simulink model "sf_demo_tl30"  (Simulink 7.5)
settings: Solver=FixedStepDiscrete  StartTime=0.0  StopTime=20  FixedStep=0.5  RelTol=1e-3
PreLoadFcn:
  | if exist('tl_preloadfcn','file'), tl_preloadfcn(gcs,101); end
PostLoadFcn:
  | if exist('tl_postloadfcn','file'), tl_postloadfcn(gcs,101); end
InitFcn:
  | if exist('tlds_init','file'), tlds_init(gcs); end
StartFcn:
  | if exist('tlds_start','file'), tlds_start(gcs); end
StopFcn:
  | if exist('tlds_stop','file'), tlds_stop(gcs); end
undefined symbols (not defined in the file or in its folder): slDataTypeAndScale
libraries: tllib x6
PreSaveFcn:
  | if exist('tl_presavefcn','file'), tl_presavefcn(gcs); end
settings Model: DS_PROJECTFILE=sf_demo_tl30.dd  TL_MAIN_DATA={'#advcodeopt',0,'codeopt',{'inliningthreshold',5,'assembler',1,'optlevel',0,'decimals',0},'frameopt',{'mexargs',''},'logopt',{'plotinterval',0.1,'globalloggingmode',4},'date',735991.66639069444}  TL_MODEL_COMMENT=This model implements a simple state machine.  TLRevision=101  Creator=rwilts  LastModifiedBy=alex  ExtModeTrigMode=oneshot  ExtModeArmWhenConnect=off  BufferReuse=off
settings DataIOCC: LimitDataPoints=off
settings OptimizationCC: BlockReduction=off  BooleanDataType=off  OptimizeBlockIOStorage=off  BufferReuse=off  ExpressionFolding=off  LocalBlockOutputs=off  InitFltsAndDblsToZero=on
settings DebuggingCC: SaveWithParameterizedLinksMsg=none  SignalResolutionControl=TryResolveAllWithWarning  SolverPrmCheckMsg=none  MultiTaskDSMMsg=warning  MultiTaskCondExecSysMsg=none
settings HardwareCC: TargetEndianess=LittleEndian  TargetHWDeviceType=MATLAB Host  ProdEqTarget=off
settings RTWCC: IncludeERTFirstTime=on
settings GRTTargetCC: TargetFcnLib=ansi_tfl_tmw.mat

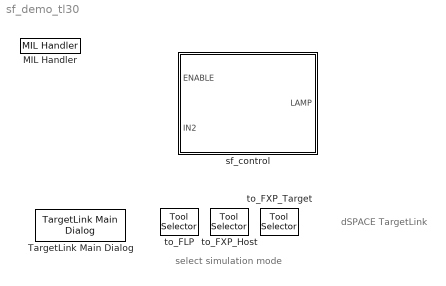
== system sf_demo_tl30 ==
  note: select simulation mode
  note: dSPACE TargetLink
  MIL Handler : tllib/MIL Handler  data={'date',735991.66638890048}
  TargetLink Main Dialog : tllib/TargetLink Main Dialog  SystemSampleTime=-1
  sf_control : Subsystem  Tag=TargetLink Simulation Frame
      settings: CopyFcn=if exist('tl_copyfcn','file'), tl_copyfcn(gcbh); end  NameChangeFcn=if exist('tl_framenamechangefcn','file'), tl_framenamechangefcn(gcbh); end
      settings: OpenFcn=|
      | if exist('open_tlsubsystem','file')
      |    open_tlsubsystem(gcbh);
      | else
      |    tlsubsystem = ...
      |       find_system(gcb, ...
      |       'LookUnderMasks','on', ...
      |       'FollowLinks','on', ...
      |       'Tag','MIL Subsystem');
      |    open_system(tlsubsystem);
      | end
      mask Type: TL_SimFrame
      mask Display: disp('TargetLink\nModel-\nin-the-loop\nmode')
  to_FLP : tllib/Tool Selector  Description=MIL\nmode  SystemSampleTime=-1  data={'date',735991.66638510418}
  to_FXP_Host : tllib/Tool Selector  Description=SIL\nmode  SystemSampleTime=-1  data={'date',735991.66638506949}
  to_FXP_Target : tllib/Tool Selector  Description=PIL\nmode  SystemSampleTime=-1  data={'date',735991.66638503468}

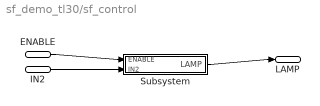
== system sf_demo_tl30/sf_control ==
  ENABLE : Inport  SampleTime=0.5  DataType=Specify via dialog  OutDataType=slDataTypeAndScale(('osc_int16'),('2^0'))  OutDataTypeStr=slDataTypeAndScale(('osc_int16'),('2^0'))
  IN2 : Inport  Port=2  SampleTime=0.5  DataType=Specify via dialog  OutDataType=osc_int16  OutDataTypeStr=osc_int16
  Subsystem : Subsystem  Tag=struct('sfcnName','sf_control_sf','subFunction','','srcSubsystem','')
      settings: OpenFcn=warndlg(get_param(gcb,'MaskHelp'),'Serious Warning');
      mask Type: TL_Enable
      mask Help: This subsystem keeps the TargetLink subsystem (subsystem with TargetLink blocks for production code generation), and is needed for the TargetLink simulation frame to work properly. DO NOT DELETE OR MODIFY IT!
  LAMP : Outport  OutDataType=sfix(16)  OutScaling=2^0
  wires:
  ENABLE/1 -> Subsystem/1(ENABLE)
  IN2/1 -> Subsystem/2(IN2)
  Subsystem/1(LAMP) -> LAMP/1

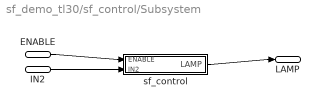
== system sf_demo_tl30/sf_control/Subsystem ==
  ENABLE : Inport  SampleTime=0.5  DataType=Specify via dialog  OutDataType=slDataTypeAndScale(('osc_int16'),('2^0'))  OutDataTypeStr=slDataTypeAndScale(('osc_int16'),('2^0'))
  IN2 : Inport  Port=2  SampleTime=0.5  DataType=Specify via dialog  OutDataType=osc_int16  OutDataTypeStr=osc_int16
  sf_control : Subsystem  Tag=MIL Subsystem  Description=a
      settings: CopyFcn=if exist('tl_copyfcn','file'), tl_copyfcn(gcbh); end  NameChangeFcn=if exist('tl_namechangefcn','file'), tl_namechangefcn(gcbh); end  DestroyFcn=if exist('update_tl_main_dlg','file'), update_tl_main_dlg('TL_subs_display'); end
      mask Display: disp('TargetLink Subsystem')
  LAMP : Outport  OutDataType=sfix(16)  OutScaling=2^0
  wires:
  ENABLE/1 -> sf_control/1(ENABLE)
  IN2/1 -> sf_control/2(IN2)
  sf_control/1(LAMP) -> LAMP/1

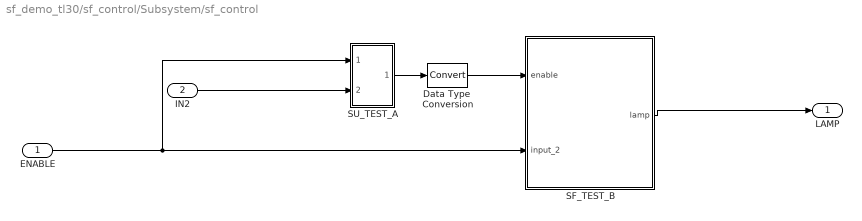
== system sf_demo_tl30/sf_control/Subsystem/sf_control ==
  ENABLE : Inport  PortDimensions=1  SampleTime=0.5  DataType=Specify via dialog  OutDataType=osc_int16  OutScaling=2^0  OutDataTypeStr=slDataTypeAndScale(('osc_int16'),('2^0'))  mask(TL_Inport){data={'logdata',{'maxnumvals',4096,'plotchannels',1,'loggingmode',1},'output',{'max',1,'min',0,'class','FCN_ARG','type','Int8'},'date',735991.66638878477}}
      settings: DeleteFcn=if exist('delete_tlblock','file')==2,delete_tlblock(gcbh);end  OpenFcn=if exist('tl_open_blockdlg','file')==2,tl_open_blockdlg(gcbh);else,open_system(gcbh,'parameter');end
      settings: CopyFcn=|
      | if exist('tl_reset_reviewflag','file')==2
      |     tl_reset_reviewflag(gcbh);
      | end
      | if exist('tl_check_ports','file')
      |     tl_check_ports(gcbh);
      | end
      settings: NameChangeFcn=|
      | if exist('rename_tlblock','file')==2,rename_tlblock(gcbh);end
      | if exist('tl_check_ports','file'), tl_check_ports(gcbh); end
      mask Help: eval(['if exist(''tl_online_help'',''file'') == 2, tl_online_help(''Topic'',''TL_Inport''),else, web([''jar:file:///'',matlabroot,''/help/toolbox/simulink/help.jar!/slref/' lower(get_param(gcbh,'Blocktype')) '.html''], ''-helpbrowser''),end'])
      mask Display: plot([0.2 0.35 NaN 0.65 0.8],[0 1 NaN 0 1]);
  IN2 : Inport  Port=2  PortDimensions=1  SampleTime=0.5  DataType=Specify via dialog  OutDataType=osc_int16  OutDataTypeStr=osc_int16  mask(TL_Inport){data={'logdata',{'maxnumvals',4096,'plotchannels',1,'loggingmode',1},'output',{'max',1,'min',0,'class','FCN_ARG','type','Int8'},'date',735991.66638833331}}
      settings: DeleteFcn=if exist('delete_tlblock','file')==2,delete_tlblock(gcbh);end  OpenFcn=if exist('tl_open_blockdlg','file')==2,tl_open_blockdlg(gcbh);else,open_system(gcbh,'parameter');end
      settings: CopyFcn=|
      | if exist('tl_reset_reviewflag','file')==2
      |     tl_reset_reviewflag(gcbh);
      | end
      | if exist('tl_check_ports','file')
      |     tl_check_ports(gcbh);
      | end
      settings: NameChangeFcn=|
      | if exist('rename_tlblock','file')==2,rename_tlblock(gcbh);end
      | if exist('tl_check_ports','file'), tl_check_ports(gcbh); end
      mask Help: eval(['if exist(''tl_online_help'',''file'') == 2, tl_online_help(''Topic'',''TL_Inport''),else, web([''jar:file:///'',matlabroot,''/help/toolbox/simulink/help.jar!/slref/' lower(get_param(gcbh,'Blocktype')) '.html''], ''-helpbrowser''),end'])
      mask Display: plot([0.2 0.35 NaN 0.65 0.8],[0 1 NaN 0 1]);
  Data Type  Conversion : DataTypeConversion  OutDataType=osc_boolean  SaturateOnIntegerOverflow=on  RndMeth=Zero
  SF_TEST_B : Stateflow chart  TreatAsAtomicUnit=on
  SU_TEST_A : Subsystem  TreatAsAtomicUnit=on
  LAMP : Outport  PortDimensions=1  DataType=int32  OutDataType=sfix(16)  OutScaling=2^0  OutDataTypeStr=int32  mask(TL_Outport){data={'logdata',{'plotchannels',1},'output',{'max',1,'min',0,'class','DISP','type','UInt8'},'autoscaling',{'mode',2},'date',735991.66638550931}}
      settings: DeleteFcn=if exist('delete_tlblock','file')==2,delete_tlblock(gcbh);end  OpenFcn=if exist('tl_open_blockdlg','file')==2,tl_open_blockdlg(gcbh);else,open_system(gcbh,'parameter');end
      settings: CopyFcn=|
      | if exist('tl_reset_reviewflag','file')==2
      |     tl_reset_reviewflag(gcbh);
      | end
      | if exist('tl_check_ports','file')
      |     tl_check_ports(gcbh);
      | end
      settings: NameChangeFcn=|
      | if exist('rename_tlblock','file')==2,rename_tlblock(gcbh);end
      | if exist('tl_check_ports','file'), tl_check_ports(gcbh); end
      mask Help: eval(['if exist(''tl_online_help'',''file'') == 2, tl_online_help(''Topic'',''TL_Outport''),else, web([''jar:file:///'',matlabroot,''/help/toolbox/simulink/help.jar!/slref/' lower(get_param(gcbh,'Blocktype')) '.html''], ''-helpbrowser''),end'])
      mask Display: plot([0.2 0.35 NaN 0.65 0.8],[0 1 NaN 0 1]);
  wires:
  SF_TEST_B/1(lamp) -> LAMP/1
  ENABLE/1 -> SU_TEST_A/1(In1), SF_TEST_B/2(input_2)
  IN2/1 -> SU_TEST_A/2(In2)
  SU_TEST_A/1(Out1) -> Data Type  Conversion/1
  Data Type  Conversion/1 -> SF_TEST_B/1(enable)

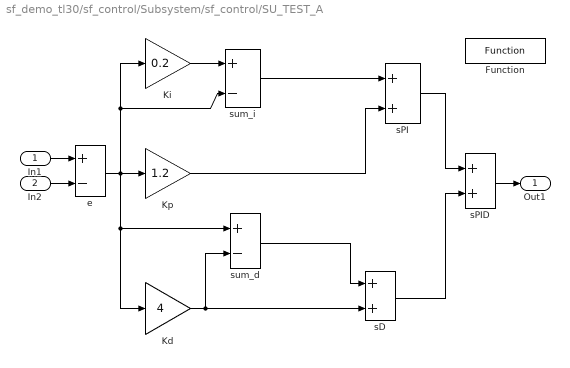
== system sf_demo_tl30/sf_control/Subsystem/sf_control/SU_TEST_A ==
  In1 : Inport  DataType=Specify via dialog  OutDataType=osc_int16  OutDataTypeStr=osc_int16
  In2 : Inport  Port=2  DataType=Specify via dialog  OutDataType=osc_int16  OutDataTypeStr=osc_int16
  Function : tllib/Function  SystemSampleTime=-1  data={'date',735991.66638493061}
  Kd : Gain  Tag="Gain block of the dSPACE Fixed Point Code Generation Environment.      \\n                                                                       \\n signal is equal to the product of the input signal and the gain value:\\n\t\ty = G u"  Description=|  Gain=4  ParameterDataType=sfix(16)  ParameterScaling=2^0  OutDataType=sfix(16)  OutScaling=2^0  OutDataTypeStr=Inherit: Inherit via back propagation  mask(TL_Gain){data={'logdata',{'plotchannels',1},'output',{'type','Int8','lsb',2^-15},'gain',{'name','P_$D','class','CAL','type','UInt8','lsb',2^-5},'date',735991.66638789349}}
      | Gain block of dSPACE TargetLink.
      | 
      | Output signal is equal to the product of the input signal and the gain value:
      |         y = G u
      settings: CopyFcn=set_param(gcb,'ReferenceBlock',''); set_param(gcb,'Tag','COPIED_DURING_UPGRADE');set_param(gcb,'CopyFcn','');  DeleteFcn=if exist('delete_tlblock','file')==2,delete_tlblock(gcbh);end  NameChangeFcn=if exist('rename_tlblock','file')==2,rename_tlblock(gcbh);end  OpenFcn=if exist('tl_open_blockdlg','file')==2,tl_open_blockdlg(gcbh);else,open_system(gcbh,'parameter');end
      mask Help: eval(['if exist(''tl_online_help'',''file'') == 2, tl_online_help(''Topic'',''TL_Gain''),else, web([''jar:file:///'',matlabroot,''/help/toolbox/simulink/help.jar!/slref/' lower(get_param(gcbh,'Blocktype')) '.html''], ''-helpbrowser''),end'])
      mask Display: plot([0, .9, 0],[.05, .5, .95])
  Ki : Gain  Description=|  Gain=0.2  ParameterDataType=sfix(16)  ParameterScaling=2^0  OutDataType=sfix(16)  OutScaling=2^0  mask(TL_Gain){data={'logdata',{'plotchannels',[]},'output',{'lsb',2^-20},'gain',{'name','P_$D','class','CAL','type','UInt8','lsb',2^-10},'date',735991.66638756939}}
      | Gain block of dSPACE TargetLink.
      | 
      | Output signal is equal to the product of the input signal and the gain value:
      |         y = G u
      settings: CopyFcn=set_param(gcb,'ReferenceBlock',''); set_param(gcb,'Tag','COPIED_DURING_UPGRADE');set_param(gcb,'CopyFcn','');  DeleteFcn=if exist('delete_tlblock','file')==2,delete_tlblock(gcbh);end  NameChangeFcn=if exist('rename_tlblock','file')==2,rename_tlblock(gcbh);end  OpenFcn=if exist('tl_open_blockdlg','file')==2,tl_open_blockdlg(gcbh);else,open_system(gcbh,'parameter');end
      mask Help: eval(['if exist(''tl_online_help'',''file'') == 2, tl_online_help(''Topic'',''TL_Gain''),else, web([''jar:file:///'',matlabroot,''/help/toolbox/simulink/help.jar!/slref/' lower(get_param(gcbh,'Blocktype')) '.html''], ''-helpbrowser''),end'])
      mask Display: plot([0, .9, 0],[.05, .5, .95])
  Kp : Gain  Tag="Gain block of the dSPACE Fixed Point Code Generation Environment.      \\n                                                                       \\n signal is equal to the product of the input signal and the gain value:\\n\t\ty = G u"  Description=|  Gain=1.2  ParameterDataType=sfix(16)  ParameterScaling=2^0  OutDataType=sfix(16)  OutScaling=2^0  mask(TL_Gain){data={'logdata',{'plotchannels',[]},'output',{'lsb',2^-17},'gain',{'name','P_$D','class','CAL','type','UInt8','lsb',2^-7},'date',735991.66638724541}}
      | Gain block of dSPACE TargetLink.
      | 
      | Output signal is equal to the product of the input signal and the gain value:
      |         y = G u
      settings: CopyFcn=set_param(gcb,'ReferenceBlock',''); set_param(gcb,'Tag','COPIED_DURING_UPGRADE');set_param(gcb,'CopyFcn','');  DeleteFcn=if exist('delete_tlblock','file')==2,delete_tlblock(gcbh);end  NameChangeFcn=if exist('rename_tlblock','file')==2,rename_tlblock(gcbh);end  OpenFcn=if exist('tl_open_blockdlg','file')==2,tl_open_blockdlg(gcbh);else,open_system(gcbh,'parameter');end
      mask Help: eval(['if exist(''tl_online_help'',''file'') == 2, tl_online_help(''Topic'',''TL_Gain''),else, web([''jar:file:///'',matlabroot,''/help/toolbox/simulink/help.jar!/slref/' lower(get_param(gcbh,'Blocktype')) '.html''], ''-helpbrowser''),end'])
      mask Display: plot([0, .9, 0],[.05, .5, .95])
  e : Sum  Description=|  Inputs=+-  OutDataType=sfix(16)  OutScaling=2^-10  mask(TL_Sum){data={'logdata',{'plotchannels',1,'loggingmode',1},'output',{'lsb',2^-18,'checkmin',1,'checkmax',1},'date',735991.666386956}}
      | Sum block of dSPACE TargetLink.
      | 
      | Output signal is equal to the sum of the input signals.
      | The list of signs is specified according to conventions for Simulink Sum blocks.
      settings: CopyFcn=set_param(gcb,'ReferenceBlock',''); set_param(gcb,'Tag','COPIED_DURING_UPGRADE');set_param(gcb,'CopyFcn','');  DeleteFcn=if exist('delete_tlblock','file')==2,delete_tlblock(gcbh);end  NameChangeFcn=if exist('rename_tlblock','file')==2,rename_tlblock(gcbh);end  OpenFcn=if exist('tl_open_blockdlg','file')==2,tl_open_blockdlg(gcbh);else,open_system(gcbh,'parameter');end
      mask Help: eval(['if exist(''tl_online_help'',''file'') == 2, tl_online_help(''Topic'',''TL_Sum''),else, web([''jar:file:///'',matlabroot,''/help/toolbox/simulink/help.jar!/slref/' lower(get_param(gcbh,'Blocktype')) '.html''], ''-helpbrowser''),end'])
      mask Display: plot([-0.05, 1.05, NaN, -0.05, 1.05],[.01, .01, NaN, .99, .99])
  sD : Sum  Tag="Sum block of the dSPACE Fixed Point Code Generation Environment.\\n                                                                \\nOutput signal is equal to the sum of the two input signals:     \\n                                                                \\n\t\ty = u1 - u2"  Description=|  OutDataType=sfix(16)  OutScaling=2^-10  OutDataTypeStr=Inherit: Inherit via back propagation  mask(TL_Sum){data={'logdata',{'plotchannels',1},'output',{'lsb',2^-15},'date',735991.66638671292}}
      | Sum block of dSPACE TargetLink.
      | 
      | Output signal is equal to the sum of the input signals.
      | The list of signs is specified according to conventions for Simulink Sum blocks.
      settings: CopyFcn=set_param(gcb,'ReferenceBlock',''); set_param(gcb,'Tag','COPIED_DURING_UPGRADE');set_param(gcb,'CopyFcn','');  DeleteFcn=if exist('delete_tlblock','file')==2,delete_tlblock(gcbh);end  NameChangeFcn=if exist('rename_tlblock','file')==2,rename_tlblock(gcbh);end  OpenFcn=if exist('tl_open_blockdlg','file')==2,tl_open_blockdlg(gcbh);else,open_system(gcbh,'parameter');end
      mask Help: eval(['if exist(''tl_online_help'',''file'') == 2, tl_online_help(''Topic'',''TL_Sum''),else, web([''jar:file:///'',matlabroot,''/help/toolbox/simulink/help.jar!/slref/' lower(get_param(gcbh,'Blocktype')) '.html''], ''-helpbrowser''),end'])
      mask Display: plot([-0.05, 1.05, NaN, -0.05, 1.05],[.01, .01, NaN, .99, .99])
  sPI : Sum  Tag="Sum block of the dSPACE Fixed Point Code Generation Environment.\\n                                                                \\nOutput signal is equal to the sum of the two input signals:     \\n                                                                \\n\t\ty = u1 - u2"  Description=|  OutDataType=sfix(16)  OutScaling=2^-10  OutDataTypeStr=Inherit: Inherit via back propagation  mask(TL_Sum){data={'logdata',{'plotchannels',[]},'output',{'lsb',2^-17},'date',735991.66638648149}}
      | Sum block of dSPACE TargetLink.
      | 
      | Output signal is equal to the sum of the input signals.
      | The list of signs is specified according to conventions for Simulink Sum blocks.
      settings: CopyFcn=set_param(gcb,'ReferenceBlock',''); set_param(gcb,'Tag','COPIED_DURING_UPGRADE');set_param(gcb,'CopyFcn','');  DeleteFcn=if exist('delete_tlblock','file')==2,delete_tlblock(gcbh);end  NameChangeFcn=if exist('rename_tlblock','file')==2,rename_tlblock(gcbh);end  OpenFcn=if exist('tl_open_blockdlg','file')==2,tl_open_blockdlg(gcbh);else,open_system(gcbh,'parameter');end
      mask Help: eval(['if exist(''tl_online_help'',''file'') == 2, tl_online_help(''Topic'',''TL_Sum''),else, web([''jar:file:///'',matlabroot,''/help/toolbox/simulink/help.jar!/slref/' lower(get_param(gcbh,'Blocktype')) '.html''], ''-helpbrowser''),end'])
      mask Display: plot([-0.05, 1.05, NaN, -0.05, 1.05],[.01, .01, NaN, .99, .99])
  sPID : Sum  Description=|  OutDataType=sfix(16)  OutScaling=2^-10  OutDataTypeStr=Inherit: Inherit via back propagation  mask(TL_Sum){data={'logdata',{'plotchannels',1},'output',{'lsb',2^-15},'date',735991.66638625006}}
      | Sum block of dSPACE TargetLink.
      | 
      | Output signal is equal to the sum of the input signals.
      | The list of signs is specified according to conventions for Simulink Sum blocks.
      settings: CopyFcn=set_param(gcb,'ReferenceBlock',''); set_param(gcb,'Tag','COPIED_DURING_UPGRADE');set_param(gcb,'CopyFcn','');  DeleteFcn=if exist('delete_tlblock','file')==2,delete_tlblock(gcbh);end  NameChangeFcn=if exist('rename_tlblock','file')==2,rename_tlblock(gcbh);end  OpenFcn=if exist('tl_open_blockdlg','file')==2,tl_open_blockdlg(gcbh);else,open_system(gcbh,'parameter');end
      mask Help: eval(['if exist(''tl_online_help'',''file'') == 2, tl_online_help(''Topic'',''TL_Sum''),else, web([''jar:file:///'',matlabroot,''/help/toolbox/simulink/help.jar!/slref/' lower(get_param(gcbh,'Blocktype')) '.html''], ''-helpbrowser''),end'])
      mask Display: plot([-0.05, 1.05, NaN, -0.05, 1.05],[.01, .01, NaN, .99, .99])
  sum_d : Sum  Description=|  Inputs=+-  OutDataType=sfix(16)  OutScaling=2^-10  OutDataTypeStr=Inherit: Inherit via back propagation  mask(TL_Sum){data={'logdata',{'plotchannels',[]},'output',{'lsb',2^-15},'date',735991.66638601851}}
      | Sum block of dSPACE TargetLink.
      | 
      | Output signal is equal to the sum of the input signals.
      | The list of signs is specified according to conventions for Simulink Sum blocks.
      settings: CopyFcn=set_param(gcb,'ReferenceBlock',''); set_param(gcb,'Tag','COPIED_DURING_UPGRADE');set_param(gcb,'CopyFcn','');  DeleteFcn=if exist('delete_tlblock','file')==2,delete_tlblock(gcbh);end  NameChangeFcn=if exist('rename_tlblock','file')==2,rename_tlblock(gcbh);end  OpenFcn=if exist('tl_open_blockdlg','file')==2,tl_open_blockdlg(gcbh);else,open_system(gcbh,'parameter');end
      mask Help: eval(['if exist(''tl_online_help'',''file'') == 2, tl_online_help(''Topic'',''TL_Sum''),else, web([''jar:file:///'',matlabroot,''/help/toolbox/simulink/help.jar!/slref/' lower(get_param(gcbh,'Blocktype')) '.html''], ''-helpbrowser''),end'])
      mask Display: plot([-0.05, 1.05, NaN, -0.05, 1.05],[.01, .01, NaN, .99, .99])
  sum_i : Sum  Tag="Sum block of the dSPACE Fixed Point Code Generation Environment.\\n                                                                \\nOutput signal is equal to the sum of the two input signals:     \\n                                                                \\n\t\ty = u1 - u2"  Description=|  Inputs=+-  OutDataType=sfix(16)  OutScaling=2^-10  mask(TL_Sum){data={'logdata',{'plotchannels',[]},'output',{'lsb',2^-19},'date',735991.66638578707}}
      | Sum block of dSPACE TargetLink.
      | 
      | Output signal is equal to the sum of the input signals.
      | The list of signs is specified according to conventions for Simulink Sum blocks.
      settings: CopyFcn=set_param(gcb,'ReferenceBlock',''); set_param(gcb,'Tag','COPIED_DURING_UPGRADE');set_param(gcb,'CopyFcn','');  DeleteFcn=if exist('delete_tlblock','file')==2,delete_tlblock(gcbh);end  NameChangeFcn=if exist('rename_tlblock','file')==2,rename_tlblock(gcbh);end  OpenFcn=if exist('tl_open_blockdlg','file')==2,tl_open_blockdlg(gcbh);else,open_system(gcbh,'parameter');end
      mask Help: eval(['if exist(''tl_online_help'',''file'') == 2, tl_online_help(''Topic'',''TL_Sum''),else, web([''jar:file:///'',matlabroot,''/help/toolbox/simulink/help.jar!/slref/' lower(get_param(gcbh,'Blocktype')) '.html''], ''-helpbrowser''),end'])
      mask Display: plot([-0.05, 1.05, NaN, -0.05, 1.05],[.01, .01, NaN, .99, .99])
  Out1 : Outport  OutDataType=sfix(16)  OutScaling=2^0
  wires:
  Kd/1 -> sum_d/2, sD/2
  sD/1 -> sPID/2
  sum_d/1 -> sD/1
  sPI/1 -> sPID/1
  sum_i/1 -> sPI/1
  Ki/1 -> sum_i/1
  Kp/1 -> sPI/2
  e/1 -> Kp/1, Ki/1, sum_i/2, Kd/1, sum_d/1
  In1/1 -> e/1
  In2/1 -> e/2
  sPID/1 -> Out1/1

== stateflow chart sf_control/Subsystem/sf_control/SF_TEST_B ==
  settings: sampleTime=1
  state do_blink
    state BLINKER_ON/
      entry:lamp=1;
    state BLINKER_OFF
      entry: lamp = 0;
    BLINKER_ON -> BLINKER_OFF
    BLINKER_OFF -> BLINKER_ON
  state OFF
    entry: lamp = 0;
  (default) -> OFF
  OFF -> BLINKER_ON : [enable == 1]
  do_blink -> OFF : [enable==0]
  data: enable input osc_boolean; lamp output osc_int32; input_2 input osc_int16
  data enable settings: description=$TL$ createinputvariable=1; $TL$
  data input_2 settings: description=$TL$ createinputvariable=1; $TL$
